simulink model "chap7_4sim"  (Simulink 7.7)
settings: Solver=ode3  StartTime=0.0  StopTime=30  FixedStep=0.001  RelTol=1e-5
settings Model: Creator=hp  LastModifiedBy=ljk  ExtModeTrigMode=oneshot  ExtModeArmWhenConnect=off
settings DataIOCC: LimitDataPoints=off  SignalLoggingName=sigsOut
settings OptimizationCC: BooleanDataType=off  InitFltsAndDblsToZero=on
settings DebuggingCC: SaveWithParameterizedLinksMsg=none  SignalResolutionControl=TryResolveAllWithWarning  SolverPrmCheckMsg=none  MultiTaskDSMMsg=warning  MultiTaskCondExecSysMsg=none  StrictBusMsg=None
settings HardwareCC: TargetUnknown=on
settings RTWCC: IncludeERTFirstTime=on
settings CodeAppCC: CustomSymbolStrType=$N$R$M_T
settings GRTTargetCC: TargetFcnLib=ansi_tfl_tmw.mat

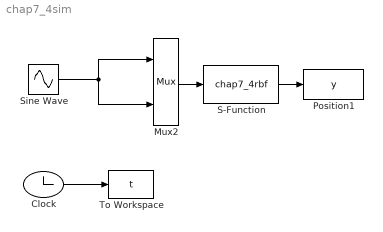
== system chap7_4sim ==
  Clock : Clock
      settings: Decimation=10
  Mux2 : Mux  Inputs=2
  Position1 : ToWorkspace  VariableName=y  SampleTime=-1  SaveFormat=Array
  S-Function : S-Function  FunctionName=chap7_4rbf  EnableBusSupport=off
  Sine Wave : Sin  SampleTime=0
  To Workspace : ToWorkspace  VariableName=t  SampleTime=-1  SaveFormat=Array
  wires:
  S-Function/1 -> Position1/1
  Clock/1 -> To Workspace/1
  Mux2/1 -> S-Function/1
  Sine Wave/1 -> Mux2/1, Mux2/2
